simulink model "SixDoFEq"  (R2020a)
settings: Solver=VariableStepAuto  StartTime=0.0  StopTime=Tfinal  FixedStep=Ts  RelTol=1e-3
undefined symbols (not defined in the file): Earth, inertia, initial, mass, WGS84
libraries: sharedtransform x2, sharedutil x2, aerolibtransform2 x1
settings Model: Creator=Fatih  LastModifiedBy=Fatih

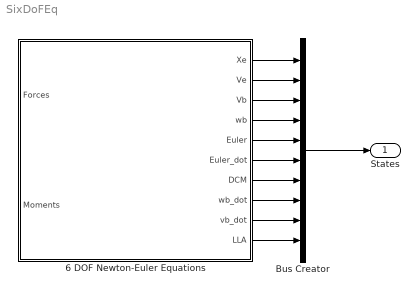
== system SixDoFEq ==
  "6 DOF Newton-Euler Equations " : Subsystem
  Bus Creator : BusCreator  Inputs=10
  States : Outport
  wires:
  "6 DOF Newton-Euler Equations "/1(Xe) -> Bus Creator/1
  "6 DOF Newton-Euler Equations "/2(Ve) -> Bus Creator/2
  "6 DOF Newton-Euler Equations "/3(Vb) -> Bus Creator/3
  "6 DOF Newton-Euler Equations "/4(wb) -> Bus Creator/4
  "6 DOF Newton-Euler Equations "/5(Euler) -> Bus Creator/5
  "6 DOF Newton-Euler Equations "/6(Euler_dot) -> Bus Creator/6
  "6 DOF Newton-Euler Equations "/7(DCM) -> Bus Creator/7
  "6 DOF Newton-Euler Equations "/8(wb_dot) -> Bus Creator/8
  "6 DOF Newton-Euler Equations "/9(vb_dot) -> Bus Creator/9
  "6 DOF Newton-Euler Equations "/10("LLA ") -> Bus Creator/10
  Bus Creator/1 -> States/1

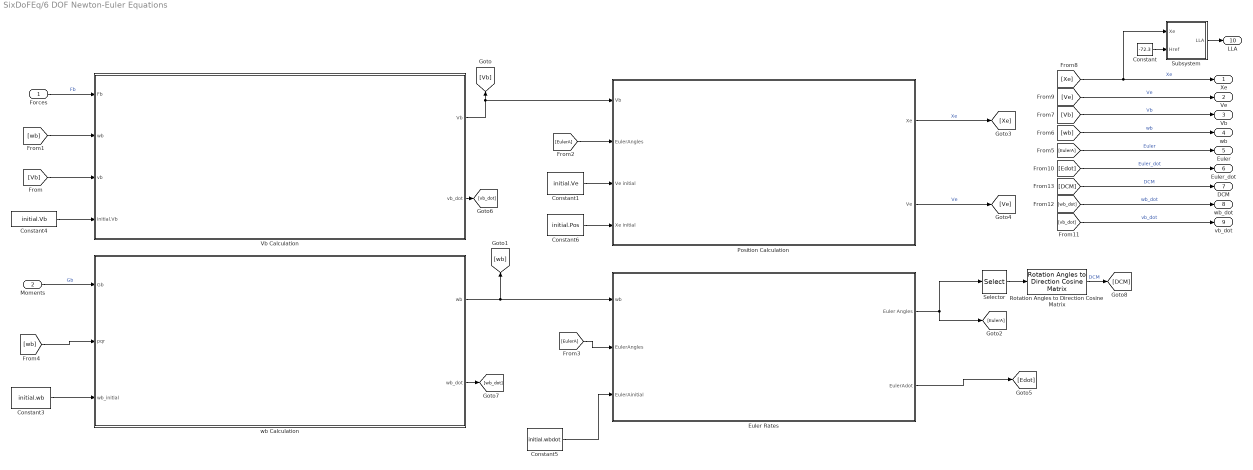
== system SixDoFEq/6 DOF Newton-Euler Equations  ==
  "Forces " : Inport
  Moments : Inport  Port=2
  Constant : Constant  Value=-72.3
  Constant1 : Constant  Value=initial.Ve
  Constant3 : Constant  Value=initial.wb
  Constant4 : Constant  Value=initial.Vb
  Constant5 : Constant  Value=initial.wbdot
  Constant6 : Constant  Value=initial.Pos
  Euler Rates : Subsystem
  "Position Calculation " : Subsystem
  Rotation Angles to Direction Cosine Matrix : sharedtransform/Rotation Angles to Direction Cosine Matrix  rotationOrder=ZYX  aMode=aMode
      settings: SourceProductBaseCode=AE,PW,MT,VE,VP
  Selector : Selector  InputPortWidth=3  IndexOptions=Index vector (dialog)  Indices=[3 2 1]  OutputSizes=1
  Subsystem : Subsystem
  Vb Calculation : Subsystem
  wb Calculation : Subsystem
  Xe : Outport
  Ve : Outport  Port=2
  Vb : Outport  Port=3
  wb : Outport  Port=4
  Euler : Outport  Port=5
  Euler_dot : Outport  Port=6
  DCM : Outport  Port=7
  wb_dot : Outport  Port=8
  vb_dot : Outport  Port=9
  "LLA " : Outport  Port=10
  wires:
  Vb Calculation/1(Vb) -> [Vb], "Position Calculation "/1(Vb)
  "Forces "/1 -> Vb Calculation/1(Fb)  "Fb"
  [wb] -> Vb Calculation/2(wb)
  [Vb] -> Vb Calculation/3("vb ")
  Constant4/1 -> Vb Calculation/4(initial.Vb)
  wb Calculation/1(wb) -> [wb], Euler Rates/1(wb)
  [wb] -> wb Calculation/2(pqr)
  Constant3/1 -> wb Calculation/3("wb_initial ")
  [EulerA] -> Euler Rates/2(EulerAngles)
  Constant5/1 -> Euler Rates/3("EulerAinitial ")
  Euler Rates/1(Euler Angles) -> Selector/1, [EulerA]
  [EulerA] -> "Position Calculation "/2(EulerAngles)
  Moments/1 -> wb Calculation/1(Gb)  "Gb"
  "Position Calculation "/1(Xe) -> [Xe]  "Xe"
  "Position Calculation "/2(Ve) -> [Ve]  "Ve"
  Constant6/1 -> "Position Calculation "/4("Xe initial ")
  Constant1/1 -> "Position Calculation "/3("Ve initial ")
  Selector/1 -> Rotation Angles to Direction Cosine Matrix/1
  Euler Rates/2("EulerAdot ") -> [Edot]
  Vb Calculation/2(vb_dot) -> [vb_dot]
  wb Calculation/2("wb_dot ") -> [wb_dot]
  [vb_dot] -> vb_dot/1  "vb_dot"
  [wb_dot] -> wb_dot/1  "wb_dot"
  [Edot] -> Euler_dot/1  "Euler_dot"
  [EulerA] -> Euler/1  "Euler"
  [wb] -> wb/1  "wb"
  [Vb] -> Vb/1  "Vb"
  [Ve] -> Ve/1  "Ve"
  [Xe] -> Subsystem/1(Xe), Xe/1  "Xe"
  Rotation Angles to Direction Cosine Matrix/1 -> [DCM]  "DCM"
  [DCM] -> DCM/1  "DCM"
  Constant/1 -> Subsystem/2(Href)
  Subsystem/1(LLA) -> "LLA "/1

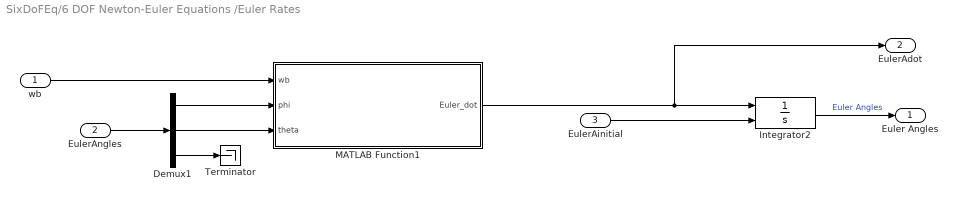
== system SixDoFEq/6 DOF Newton-Euler Equations /Euler Rates ==
  wb : Inport
  EulerAngles : Inport  Port=2
  "EulerAinitial " : Inport  Port=3
  Demux1 : Demux  Outputs=3
  Integrator2 : Integrator  InitialConditionSource=external  LimitOutput=on  UpperSaturationLimit=[pi; pi/2;pi]  LowerSaturationLimit=[-pi;-pi/2 ;-pi]  WrappedStateUpperValue=[pi; pi/2;pi]  WrappedStateLowerValue=[-pi;-pi/2 ;-pi]  IgnoreLimit=on
  MATLAB Function1 : MATLAB Function  TreatAsAtomicUnit=on
  Terminator : Terminator
  Euler Angles : Outport
  "EulerAdot " : Outport  Port=2
  wires:
  Demux1/3 -> Terminator/1
  Integrator2/1 -> Euler Angles/1  "Euler Angles"
  Demux1/2 -> MATLAB Function1/3(theta)
  Demux1/1 -> MATLAB Function1/2(phi)
  wb/1 -> MATLAB Function1/1(wb)
  "EulerAinitial "/1 -> Integrator2/2
  EulerAngles/1 -> Demux1/1
  MATLAB Function1/1(Euler_dot) -> Integrator2/1, "EulerAdot "/1

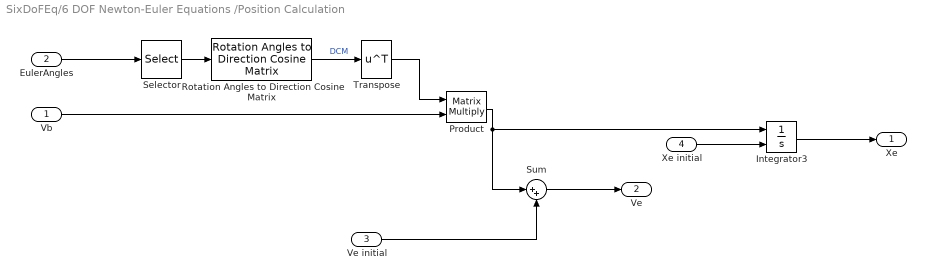
== system SixDoFEq/6 DOF Newton-Euler Equations /Position Calculation  ==
  Vb : Inport
  EulerAngles : Inport  Port=2
  "Ve initial " : Inport  Port=3
  "Xe initial " : Inport  Port=4
  Integrator3 : Integrator  InitialConditionSource=external
  Product : Product  Multiplication=Matrix(*)
  Rotation Angles to Direction Cosine Matrix : sharedtransform/Rotation Angles to Direction Cosine Matrix  rotationOrder=ZYX  aMode=aMode
      settings: SourceProductBaseCode=AE,PW,MT,VE,VP
  Selector : Selector  InputPortWidth=3  IndexOptions=Index vector (dialog)  Indices=[3 2 1]  OutputSizes=1
  Sum : Sum  Inputs=|++
  Transpose : Math  Operator=transpose  SaturateOnIntegerOverflow=on
  Xe : Outport
  Ve : Outport  Port=2
  wires:
  Product/1 -> Sum/1, Integrator3/1
  EulerAngles/1 -> Selector/1
  "Xe initial "/1 -> Integrator3/2
  Integrator3/1 -> Xe/1
  Sum/1 -> Ve/1
  "Ve initial "/1 -> Sum/2
  Selector/1 -> Rotation Angles to Direction Cosine Matrix/1
  Rotation Angles to Direction Cosine Matrix/1 -> Transpose/1  "DCM"
  Transpose/1 -> Product/1
  Vb/1 -> Product/2

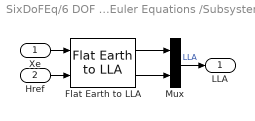
== system SixDoFEq/6 DOF Newton-Euler Equations /Subsystem ==
  Xe : Inport
  Href : Inport  Port=2
  Flat Earth to LLA : aerolibtransform2/Flat Earth to LLA  units=Metric (MKS)  ptype=Earth (WGS84)  F=1/298.257223563  R=6378137  LL0=[0 10]  psi=0
  Mux : Mux  Inputs=2
  LLA : Outport
  wires:
  Xe/1 -> Flat Earth to LLA/1
  Href/1 -> Flat Earth to LLA/2
  Flat Earth to LLA/1 -> Mux/1
  Flat Earth to LLA/2 -> Mux/2
  Mux/1 -> LLA/1  "LLA"

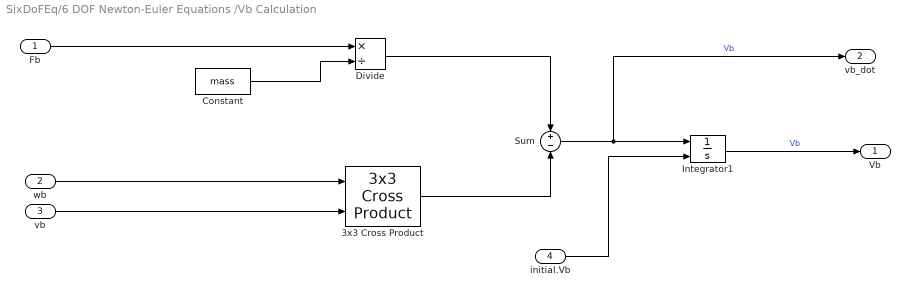
== system SixDoFEq/6 DOF Newton-Euler Equations /Vb Calculation ==
  Fb : Inport
  wb : Inport  Port=2
  "vb " : Inport  Port=3
  initial.Vb : Inport  Port=4
  3x3 Cross Product : sharedutil/3x3 Cross Product  aMode=aMode
      settings: SourceProductBaseCode=AE,PW,MT,VE,VP
  Constant : Constant  Value=mass
  Divide : Product  Inputs=*/
  Integrator1 : Integrator  InitialConditionSource=external
  Sum : Sum  Inputs=+|-
  Vb : Outport
  vb_dot : Outport  Port=2
  wires:
  3x3 Cross Product/1 -> Sum/2
  wb/1 -> 3x3 Cross Product/1
  Fb/1 -> Divide/1
  Constant/1 -> Divide/2
  Divide/1 -> Sum/1
  Integrator1/1 -> Vb/1  "Vb"
  "vb "/1 -> 3x3 Cross Product/2
  Sum/1 -> vb_dot/1, Integrator1/1  "Vb"
  initial.Vb/1 -> Integrator1/2

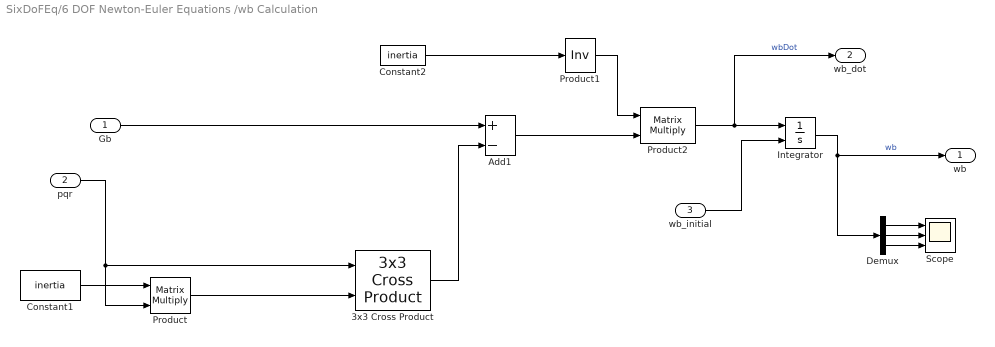
== system SixDoFEq/6 DOF Newton-Euler Equations /wb Calculation ==
  Gb : Inport
  pqr : Inport  Port=2
  "wb_initial " : Inport  Port=3
  3x3 Cross Product : sharedutil/3x3 Cross Product  aMode=aMode
      settings: SourceProductBaseCode=AE,PW,MT,VE,VP
  Add1 : Sum  Inputs=+-
  Constant1 : Constant  Value=inertia
  Constant2 : Constant  Value=inertia
  Demux : Demux  Outputs=3
  Integrator : Integrator  InitialConditionSource=external
  Product : Product  Multiplication=Matrix(*)
  Product1 : Product  Inputs=/  Multiplication=Matrix(*)
  Product2 : Product  Multiplication=Matrix(*)
  Scope : Scope  NumInputPorts=3
  wb : Outport
  "wb_dot " : Outport  Port=2
  wires:
  "wb_initial "/1 -> Integrator/2
  Add1/1 -> Product2/2
  3x3 Cross Product/1 -> Add1/2
  Integrator/1 -> wb/1, Demux/1  "wb"
  Gb/1 -> Add1/1
  Demux/1 -> Scope/1
  Demux/2 -> Scope/2
  Demux/3 -> Scope/3
  Constant2/1 -> Product1/1
  Product2/1 -> Integrator/1, "wb_dot "/1  "wbDot"
  Product1/1 -> Product2/1
  Constant1/1 -> Product/1
  pqr/1 -> Product/2, 3x3 Cross Product/1
  Product/1 -> 3x3 Cross Product/2

== matlab function SixDoFEq/6 DOF Newton-Euler Equations /Euler Rates/MATLAB Function1 ==
  data: wb input; phi input; theta input; Euler_dot output
function Euler_dot = EulerRates(wb,phi,theta)

RMatrix = [1 0 -sin(theta);...
    0 cos(phi) sin(phi)*cos(theta);...
    0 -sin(phi) cos(phi)*cos(theta)];

Euler_dot = inv(RMatrix) * wb;
end
